simulink model "SimpleSineModel"  (R2023a)
settings: Solver=VariableStepAuto  StartTime=0.0  StopTime=20  RelTol=1e-3
settings Model: Creator=MY PC  LastModifiedBy=MY PC

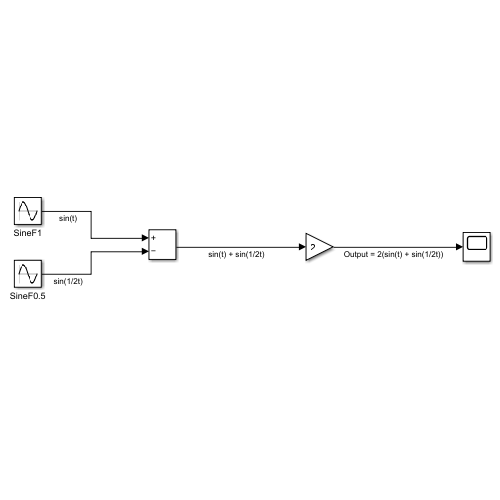
[thumbnail: Simulink's stored preview of the top-level diagram]
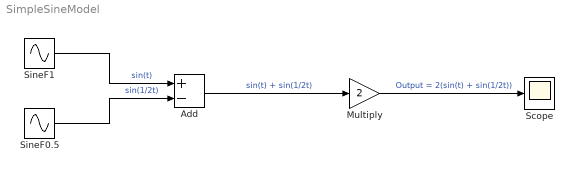
== system SimpleSineModel ==
  Add : Sum  Inputs=+-
  Multiply : Gain  Gain=2
  Scope : Scope
  SineF0.5 : Sin  Frequency=0.5  SampleTime=0
  SineF1 : Sin  SampleTime=0
  wires:
  SineF1/1 -> Add/1  "sin(t)"
  SineF0.5/1 -> Add/2  "sin(1/2t)"
  Add/1 -> Multiply/1  "sin(t) + sin(1/2t)"
  Multiply/1 -> Scope/1  "Output = 2(sin(t) + sin(1/2t))"
